simulink model "eha_model_w_svsf"  (R2015b)
settings: Solver=ode4  StartTime=0.0  StopTime=20  FixedStep=0.01  RelTol=1e-3
values from neighbouring files (symbols this model uses):
  A = [ 1 0.001 0; 0 1 0.001; -557.02 -28616 0.9418]    [eha_w_kalman_filter.m]
  B = [0 0 557.02]    [eha_w_kalman_filter.m]
undefined symbols (not defined in the file or in its folder): C, x0
settings Model: Creator=mathi  LastModifiedBy=Nicholas

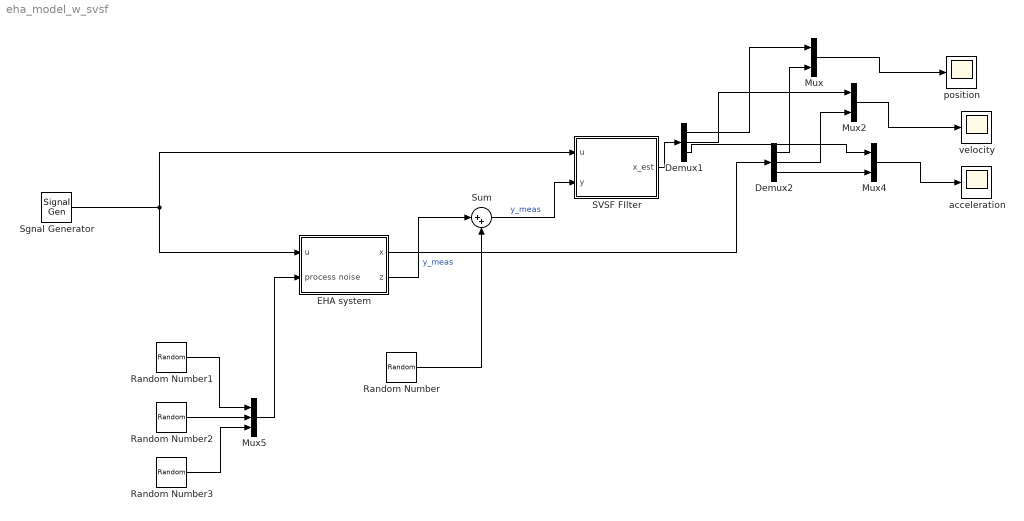
== system eha_model_w_svsf ==
  Demux1 : Demux  Outputs=3
  Demux2 : Demux  Outputs=3
  EHA system : Subsystem
  Mux : Mux  Inputs=2
  Mux2 : Mux  Inputs=2
  Mux4 : Mux  Inputs=2
  Mux5 : Mux  Inputs=3
  Random Number : RandomNumber  Variance=0.1  SampleTime=0.01
  Random Number1 : RandomNumber  Variance=0.01  SampleTime=0.01
  Random Number2 : RandomNumber  SampleTime=0.01
  Random Number3 : RandomNumber  Variance=10  SampleTime=0.01
  SVSF FIlter : Subsystem
  Sgnal Generator : SignalGenerator  WaveForm=square  Units=rad/sec
  Sum : Sum  Inputs=|++
  acceleration : Scope
  position : Scope
  velocity : Scope
  wires:
  Sgnal Generator/1 -> SVSF FIlter/1(u), EHA system/1(u)
  EHA system/2(z) -> Sum/1  "y_meas"
  Sum/1 -> SVSF FIlter/2(y)  "y_meas"
  Random Number/1 -> Sum/2
  SVSF FIlter/1(x_est) -> Demux1/1
  EHA system/1(x) -> Demux2/1
  Demux1/1 -> Mux/1
  Demux2/1 -> Mux/2
  Mux/1 -> position/1
  Demux1/2 -> Mux2/1
  Demux2/2 -> Mux2/2
  Mux2/1 -> velocity/1
  Demux1/3 -> Mux4/1
  Demux2/3 -> Mux4/2
  Mux4/1 -> acceleration/1
  Random Number1/1 -> Mux5/1
  Random Number2/1 -> Mux5/2
  Random Number3/1 -> Mux5/3
  Mux5/1 -> EHA system/2(process noise)

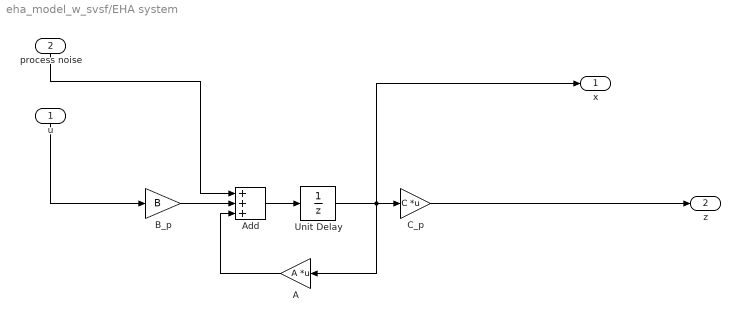
== system eha_model_w_svsf/EHA system ==
  u : Inport
  process noise : Inport  Port=2
  A : Gain  Gain=A  Multiplication=Matrix(K*u)
  Add : Sum  Inputs=+++
  B_p : Gain  Gain=B
  C_p : Gain  Gain=C  Multiplication=Matrix(K*u)
  Unit Delay : UnitDelay  InitialCondition=x0  SampleTime=-1
  x : Outport
  z : Outport  Port=2
  wires:
  Unit Delay/1 -> C_p/1, x/1, A/1
  C_p/1 -> z/1
  u/1 -> B_p/1
  Add/1 -> Unit Delay/1
  B_p/1 -> Add/2
  A/1 -> Add/3
  process noise/1 -> Add/1

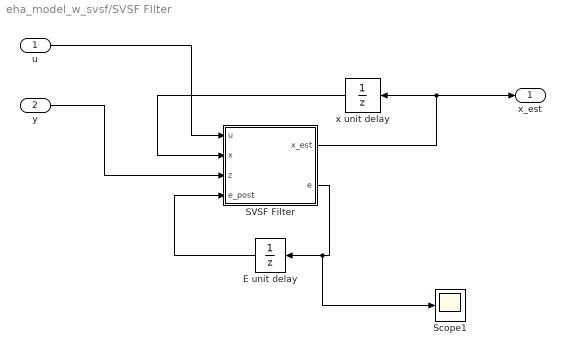
== system eha_model_w_svsf/SVSF FIlter ==
  u : Inport
  y : Inport  Port=2
  E unit delay : UnitDelay  SampleTime=-1
  SVSF Filter : MATLAB Function  TreatAsAtomicUnit=on
  Scope1 : Scope
  x unit delay : UnitDelay  InitialCondition=x0  SampleTime=-1
  x_est : Outport
  wires:
  SVSF Filter/2(e) -> Scope1/1, E unit delay/1
  E unit delay/1 -> SVSF Filter/4(e_post)
  SVSF Filter/1(x_est) -> x_est/1, x unit delay/1
  u/1 -> SVSF Filter/1(u)
  y/1 -> SVSF Filter/3(z)
  x unit delay/1 -> SVSF Filter/2(x)

== matlab function eha_model_w_svsf/SVSF FIlter/SVSF Filter ==
  data: u input; x_est output; x input; z input; e_post input; e output
function [x_est, e] = fcn(u,x,z,e_post)
%#codegen

A = [ 1 0.001 0; 0 1 0.001; -557.02 -28.616 0.9418];
B = [0 0 557.02]';
H = [1 0 0];
psi = 200;
gamma = 0.2;

%%Prediciton
x_next = A*x + B*u;

%%Update
e_priori = z - H*x_next;
if (abs(e_priori/psi) <= 1)
    sat_func = e_priori/psi;
else
    sat_func = sign(e_priori/psi);
end

K = pinv(H)*abs(abs(e_priori)+gamma*abs(e_post))*sat_func;
x_est = x_next + K;
e = z-H*x_est;
